simulink library "Lib_PFSys_GenericRectifier_TMATS"  (R2019b)
settings: Solver=ode45  StartTime=0.0  StopTime=10.0  RelTol=1e-3  EnableMultiTasking=on
Description:
  | Thomas Modules
settings Model: Creator=jwchapm2  LastModifiedBy=mebell
settings DataIOCC: LimitDataPoints=on  SaveFormat=Array  ReturnWorkspaceOutputs=off
settings OptimizationCC: ExpressionDepthLimit=2147483647  LifeSpan=inf
settings DebuggingCC: UnderspecifiedInitializationDetection=Classic  MergeDetectMultiDrivingBlocksExec=none  SolverPrmCheckMsg=warning  StateNameClashWarn=warning  SFUnexpectedBacktrackingDiag=warning  SFNoUnconditionalDefaultTransitionDiag=warning  SFExecutionAtInitializationDiag=none  ArithmeticOperatorsInVariantConditions=warning
settings HardwareCC: ProdBitPerPointer=32  ProdBitPerSizeT=32  ProdBitPerPtrDiffT=32  ProdLargestAtomicFloat=None  ProdIntDivRoundTo=Undefined  ProdEndianess=Unspecified  ProdWordSize=32  ProdHWDeviceType=32-bit Generic
settings ModelReferenceCC: PropagateSignalLabelsOutOfModel=off
settings SFSimCC: SimUseLocalCustomCode=off  CustomCodeUndefinedFunction=UseInterfaceOnly
settings RTWCC: RTWUseLocalCustomCode=off
settings CodeAppCC: StateflowObjectComments=on
settings GRTTargetCC: TargetLangStandard=C89/C90 (ANSI)  GeneratePreprocessorConditionals=Disable all
settings ConfigComp: CovMetricSettings=dw  CovHtmlReporting=on  CovSaveCumulativeToWorkspaceVar=on  CovSaveSingleToWorkspaceVar=on  CovExternalEMLEnable=off

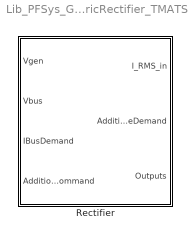
== system Lib_PFSys_GenericRectifier_TMATS ==
  Rectifier : Subsystem  mask(Motor){Eff_M=.98}
      mask prompts: Eff_M "Eff_M - Rectifier Efficiency"
      mask help:
      | This block represents a generic motor with a purely resistive input
      | impedance, and a lumped efficiency/loss model, specified as a lookup table.

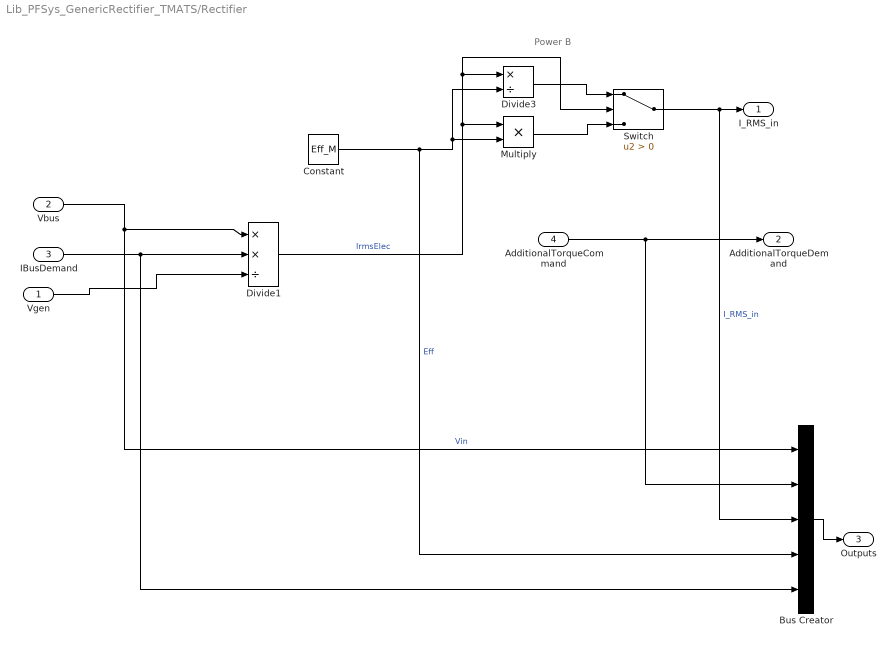
== system Lib_PFSys_GenericRectifier_TMATS/Rectifier ==
  note: Power B
  "Vgen " : Inport
  Vbus : Inport  Port=2
  IBusDemand : Inport  Port=3
  AdditionalTorqueCommand : Inport  Port=4
  Bus Creator : BusCreator  Inputs=5
  Constant : Constant  Value=Eff_M
  Divide1 : Product  Inputs=**/
  Divide3 : Product  Inputs=*/
  Multiply : Product
  Switch : Switch  Criteria=u2 > Threshold
  I_RMS_in : Outport  VectorParamsAs1DForOutWhenUnconnected=off
  AdditionalTorqueDemand : Outport  Port=2
  Outputs : Outport  Port=3  VectorParamsAs1DForOutWhenUnconnected=off
  wires:
  Bus Creator/1 -> Outputs/1
  Vbus/1 -> Divide1/1, Bus Creator/1  "Vin"
  IBusDemand/1 -> Bus Creator/5, Divide1/2
  "Vgen "/1 -> Divide1/3
  Divide1/1 -> Switch/2, Divide3/1, Multiply/1  "IrmsElec"
  Constant/1 -> Bus Creator/4, Divide3/2, Multiply/2  "Eff"
  Multiply/1 -> Switch/3
  Divide3/1 -> Switch/1
  Switch/1 -> Bus Creator/3, I_RMS_in/1  "I_RMS_in"
  AdditionalTorqueCommand/1 -> Bus Creator/2, AdditionalTorqueDemand/1
